simulink model "subsystems"  (R2023b)
settings: Solver=FixedStepAuto  StartTime=0.0  StopTime=10.0  FixedStep=1e-3  RelTol=1e-3
libraries: simulink x5
settings Model: Creator=DELL  LastModifiedBy=DELL

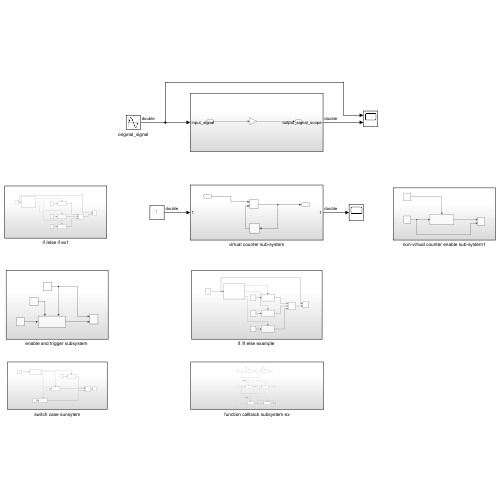
[thumbnail: Simulink's stored preview of the top-level diagram]
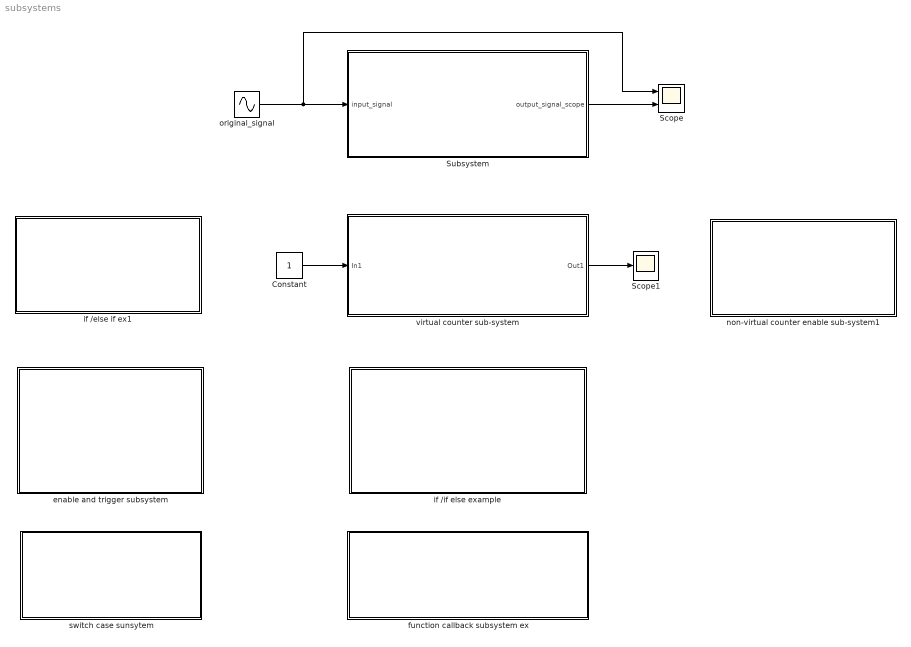
== system subsystems ==
  Constant : Constant
  Scope : Scope  NumInputPorts=2
  Scope1 : Scope
  Subsystem : Subsystem
  "enable and trigger subsystem " : Subsystem
  function callback subsystem ex : Subsystem
  if /else if ex1 : Subsystem
  "if /if else example " : Subsystem
  non-virtual counter enable sub-system1 : Subsystem
  original_signal : Sin  SampleTime=0
  switch case sunsytem : Subsystem
  virtual counter sub-system : Subsystem
  wires:
  original_signal/1 -> Subsystem/1(input_signal), Scope/1
  Subsystem/1(output_signal_scope) -> Scope/2
  Constant/1 -> virtual counter sub-system/1(In1)
  virtual counter sub-system/1(Out1) -> Scope1/1

== system subsystems/Subsystem ==
  input_signal : Inport
  Gain : Gain  Gain=2
  output_signal_scope : Outport
  wires:
  input_signal/1 -> Gain/1
  Gain/1 -> output_signal_scope/1

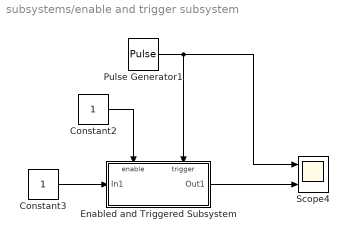
== system subsystems/enable and trigger subsystem  ==
  Constant2 : Constant
  Constant3 : Constant
  Enabled and Triggered Subsystem : Subsystem  TreatAsAtomicUnit=on
  Pulse Generator1 : DiscretePulseGenerator  PulseType=Time based  PulseWidth=50
  Scope4 : Scope  NumInputPorts=2
  wires:
  Pulse Generator1/1 -> Enabled and Triggered Subsystem/Trigger, Scope4/1
  Constant3/1 -> Enabled and Triggered Subsystem/1(In1)
  Constant2/1 -> Enabled and Triggered Subsystem/Enable
  Enabled and Triggered Subsystem/1(Out1) -> Scope4/2

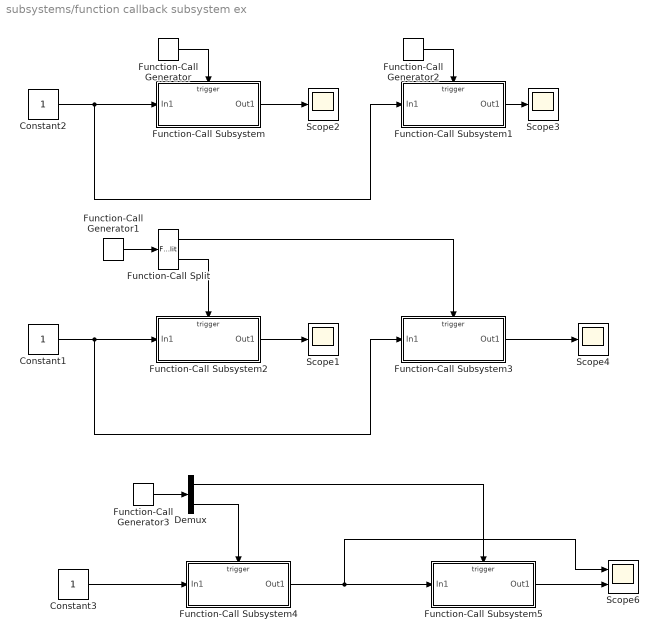
== system subsystems/function callback subsystem ex ==
  Constant1 : Constant
  Constant2 : Constant
  Constant3 : Constant
  Demux : Demux  Outputs=2
  Function-Call Generator : simulink/Ports & Subsystems/Function-Call Generator  sample_time=0.25  numberOfIterations=1  DisallowWideOutput=off
  Function-Call Generator1 : simulink/Ports & Subsystems/Function-Call Generator  sample_time=0.25  numberOfIterations=1  DisallowWideOutput=off
  Function-Call Generator2 : simulink/Ports & Subsystems/Function-Call Generator  sample_time=0.25  numberOfIterations=1  DisallowWideOutput=off
  Function-Call Generator3 : simulink/Ports & Subsystems/Function-Call Generator  sample_time=1  numberOfIterations=1  DisallowWideOutput=off
  Function-Call Split : FunctionCallSplit  IconShape=distinctive  NumOutputPorts=2  OutputPortLayout=default
  Function-Call Subsystem : Subsystem  TreatAsAtomicUnit=on
  Function-Call Subsystem1 : Subsystem  TreatAsAtomicUnit=on
  Function-Call Subsystem2 : Subsystem  TreatAsAtomicUnit=on
  Function-Call Subsystem3 : Subsystem  TreatAsAtomicUnit=on
  Function-Call Subsystem4 : Subsystem  TreatAsAtomicUnit=on
  Function-Call Subsystem5 : Subsystem  TreatAsAtomicUnit=on
  Scope{1..4} (4 alike) : Scope
  Scope6 : Scope  NumInputPorts=2
  wires:
  Function-Call Subsystem/1(Out1) -> Scope2/1
  Function-Call Generator/1 -> Function-Call Subsystem/Trigger
  Constant2/1 -> Function-Call Subsystem1/1(In1), Function-Call Subsystem/1(In1)
  Function-Call Subsystem1/1(Out1) -> Scope3/1
  Function-Call Generator2/1 -> Function-Call Subsystem1/Trigger
  Function-Call Subsystem3/1(Out1) -> Scope4/1
  Constant1/1 -> Function-Call Subsystem2/1(In1), Function-Call Subsystem3/1(In1)
  Function-Call Subsystem2/1(Out1) -> Scope1/1
  Function-Call Generator1/1 -> Function-Call Split/1
  Function-Call Split/2 -> Function-Call Subsystem2/Trigger
  Function-Call Split/1 -> Function-Call Subsystem3/Trigger
  Demux/1 -> Function-Call Subsystem5/Trigger
  Demux/2 -> Function-Call Subsystem4/Trigger
  Function-Call Generator3/1 -> Demux/1
  Function-Call Subsystem4/1(Out1) -> Function-Call Subsystem5/1(In1), Scope6/1
  Constant3/1 -> Function-Call Subsystem4/1(In1)
  Function-Call Subsystem5/1(Out1) -> Scope6/2

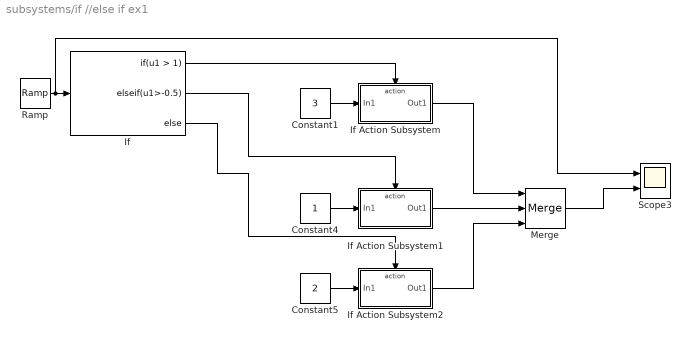
== system subsystems/if //else if ex1 ==
  Constant1 : Constant  Value=3
  Constant4 : Constant
  Constant5 : Constant  Value=2
  If : If  IfExpression=u1 > 1  ElseIfExpressions=u1>-0.5
  If Action Subsystem : Subsystem  TreatAsAtomicUnit=on
  If Action Subsystem1 : Subsystem  TreatAsAtomicUnit=on
  If Action Subsystem2 : Subsystem  TreatAsAtomicUnit=on
  Merge : Merge  Inputs=3
  Ramp : simulink/Sources/Ramp  slope=1  start=0  InitialOutput=-0.5
  Scope3 : Scope  NumInputPorts=2
  wires:
  If Action Subsystem/1(Out1) -> Merge/1
  Ramp/1 -> Scope3/1, If/1
  If/1 -> If Action Subsystem/Action
  Constant4/1 -> If Action Subsystem1/1(In1)
  Merge/1 -> Scope3/2
  If Action Subsystem2/1(Out1) -> Merge/3
  If/3 -> If Action Subsystem2/Action
  If/2 -> If Action Subsystem1/Action
  Constant1/1 -> If Action Subsystem/1(In1)
  Constant5/1 -> If Action Subsystem2/1(In1)
  If Action Subsystem1/1(Out1) -> Merge/2

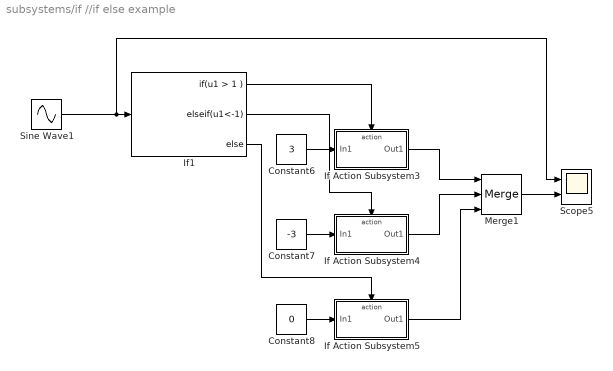
== system subsystems/if //if else example  ==
  Constant6 : Constant  Value=3
  Constant7 : Constant  Value=-3
  Constant8 : Constant  Value=0
  If Action Subsystem3 : Subsystem  TreatAsAtomicUnit=on
  If Action Subsystem4 : Subsystem  TreatAsAtomicUnit=on
  If Action Subsystem5 : Subsystem  TreatAsAtomicUnit=on
  If1 : If  IfExpression=u1 > 1  ElseIfExpressions=u1<-1
  Merge1 : Merge  Inputs=3
  Scope5 : Scope  NumInputPorts=2
  Sine Wave1 : Sin  Amplitude=7  SampleTime=0
  wires:
  If1/1 -> If Action Subsystem3/Action
  If Action Subsystem3/1(Out1) -> Merge1/1
  Merge1/1 -> Scope5/2
  If1/2 -> If Action Subsystem4/Action
  If Action Subsystem4/1(Out1) -> Merge1/2
  Constant7/1 -> If Action Subsystem4/1(In1)
  Sine Wave1/1 -> Scope5/1, If1/1
  Constant6/1 -> If Action Subsystem3/1(In1)
  Constant8/1 -> If Action Subsystem5/1(In1)
  If Action Subsystem5/1(Out1) -> Merge1/3
  If1/3 -> If Action Subsystem5/Action

== system subsystems/non-virtual counter enable sub-system1 ==
  Pulse Generator : DiscretePulseGenerator  PulseType=Time based  Period=1  PulseWidth=50
  Scope2 : Scope  NumInputPorts=2
  Sine Wave : Sin  SampleTime=0
  non-virtual counter enable sub-system : Subsystem  TreatAsAtomicUnit=on
  wires:
  Sine Wave/1 -> Scope2/2, non-virtual counter enable sub-system/1(In1)
  Pulse Generator/1 -> non-virtual counter enable sub-system/Enable
  non-virtual counter enable sub-system/1(Out1) -> Scope2/1

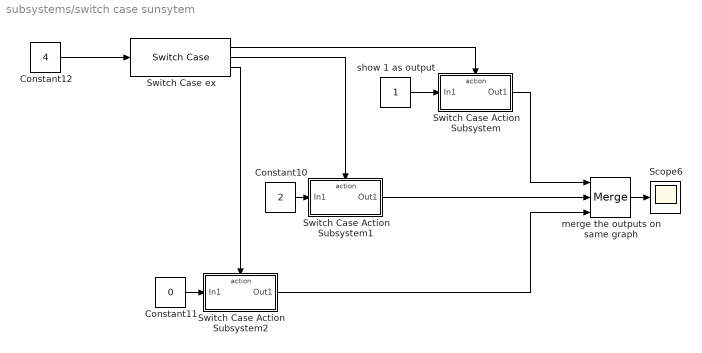
== system subsystems/switch case sunsytem ==
  Constant10 : Constant  Value=2
  Constant11 : Constant  Value=0
  Constant12 : Constant  Value=4
  Scope6 : Scope
  Switch Case Action Subsystem : Subsystem  TreatAsAtomicUnit=on
  Switch Case Action Subsystem1 : Subsystem  TreatAsAtomicUnit=on
  Switch Case Action Subsystem2 : Subsystem  TreatAsAtomicUnit=on
  Switch Case ex : SwitchCase  CaseConditions={1,[2,3,5]}
  "merge the outputs on same graph " : Merge  Inputs=3
  "show 1 as output " : Constant
  wires:
  Constant12/1 -> Switch Case ex/1
  Switch Case Action Subsystem1/1(Out1) -> "merge the outputs on same graph "/2
  Switch Case ex/2 -> Switch Case Action Subsystem1/Action
  "show 1 as output "/1 -> Switch Case Action Subsystem/1(In1)
  Switch Case ex/3 -> Switch Case Action Subsystem2/Action
  Switch Case ex/1 -> Switch Case Action Subsystem/Action
  Constant11/1 -> Switch Case Action Subsystem2/1(In1)
  Switch Case Action Subsystem/1(Out1) -> "merge the outputs on same graph "/1
  "merge the outputs on same graph "/1 -> Scope6/1
  Constant10/1 -> Switch Case Action Subsystem1/1(In1)
  Switch Case Action Subsystem2/1(Out1) -> "merge the outputs on same graph "/3

== system subsystems/virtual counter sub-system ==
  In1 : Inport
  Add : Sum
  Unit Delay : UnitDelay  SampleTime=-1  HasFrameUpgradeWarning=on
  Out1 : Outport
  wires:
  Add/1 -> Out1/1, Unit Delay/1
  Unit Delay/1 -> Add/2
  In1/1 -> Add/1

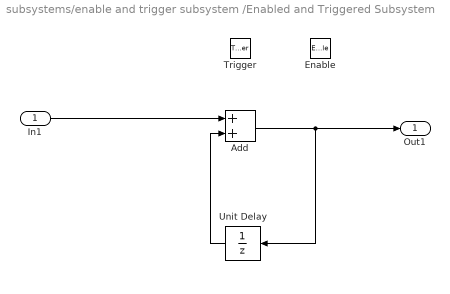
== system subsystems/enable and trigger subsystem /Enabled and Triggered Subsystem ==
  In1 : Inport
  Enable : EnablePort
  Trigger : TriggerPort  TriggerType=either  VariantControl=(inherit)
  Add : Sum
  Unit Delay : UnitDelay  SampleTime=-1  HasFrameUpgradeWarning=on
  Out1 : Outport
  wires:
  In1/1 -> Add/1
  Unit Delay/1 -> Add/2
  Add/1 -> Unit Delay/1, Out1/1

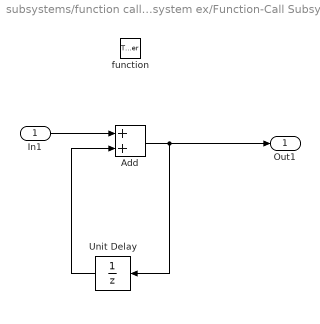
== system subsystems/function callback subsystem ex/Function-Call Subsystem ==
  In1 : Inport
  function : TriggerPort  TriggerType=function-call  VariantControl=(inherit)
  Add : Sum
  Unit Delay : UnitDelay  SampleTime=-1  HasFrameUpgradeWarning=on
  Out1 : Outport
  wires:
  In1/1 -> Add/1
  Unit Delay/1 -> Add/2
  Add/1 -> Unit Delay/1, Out1/1

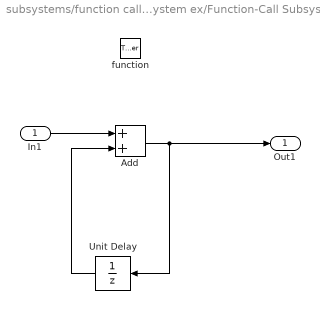
== system subsystems/function callback subsystem ex/Function-Call Subsystem1 ==
  In1 : Inport
  function : TriggerPort  TriggerType=function-call  VariantControl=(inherit)
  Add : Sum
  Unit Delay : UnitDelay  SampleTime=-1  HasFrameUpgradeWarning=on
  Out1 : Outport
  wires:
  Add/1 -> Out1/1, Unit Delay/1
  Unit Delay/1 -> Add/2
  In1/1 -> Add/1

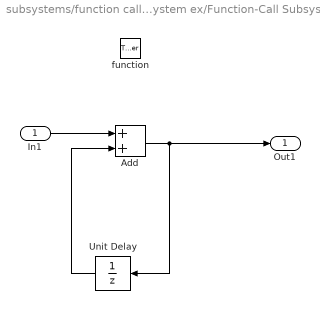
== system subsystems/function callback subsystem ex/Function-Call Subsystem2 ==
  In1 : Inport
  function : TriggerPort  TriggerType=function-call  VariantControl=(inherit)
  Add : Sum
  Unit Delay : UnitDelay  SampleTime=-1  HasFrameUpgradeWarning=on
  Out1 : Outport
  wires:
  Add/1 -> Out1/1, Unit Delay/1
  Unit Delay/1 -> Add/2
  In1/1 -> Add/1

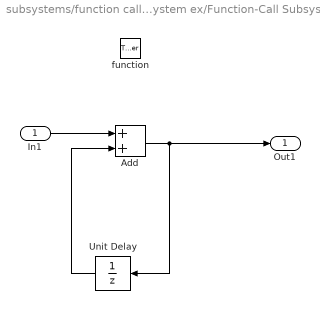
== system subsystems/function callback subsystem ex/Function-Call Subsystem3 ==
  In1 : Inport
  function : TriggerPort  TriggerType=function-call  VariantControl=(inherit)
  Add : Sum
  Unit Delay : UnitDelay  SampleTime=-1  HasFrameUpgradeWarning=on
  Out1 : Outport
  wires:
  In1/1 -> Add/1
  Unit Delay/1 -> Add/2
  Add/1 -> Unit Delay/1, Out1/1

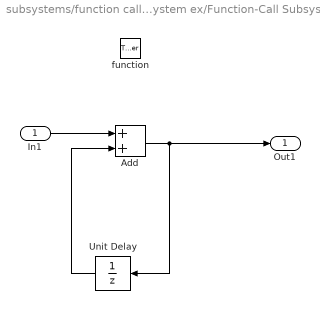
== system subsystems/function callback subsystem ex/Function-Call Subsystem4 ==
  In1 : Inport
  function : TriggerPort  TriggerType=function-call  VariantControl=(inherit)
  Add : Sum
  Unit Delay : UnitDelay  SampleTime=-1  HasFrameUpgradeWarning=on
  Out1 : Outport
  wires:
  In1/1 -> Add/1
  Unit Delay/1 -> Add/2
  Add/1 -> Unit Delay/1, Out1/1

== system subsystems/function callback subsystem ex/Function-Call Subsystem5 ==
  In1 : Inport
  function : TriggerPort  TriggerType=function-call  VariantControl=(inherit)
  Add : Sum
  Unit Delay : UnitDelay  SampleTime=-1  HasFrameUpgradeWarning=on
  Out1 : Outport
  wires:
  Add/1 -> Out1/1, Unit Delay/1
  Unit Delay/1 -> Add/2
  In1/1 -> Add/1

== system subsystems/if //else if ex1/If Action Subsystem ==
  In1 : Inport
  Action Port : ActionPort  ActionPortLabel=if(u1 > 1)
  Out1 : Outport
  wires:
  In1/1 -> Out1/1

== system subsystems/if //else if ex1/If Action Subsystem1 ==
  In1 : Inport
  Action Port : ActionPort  ActionPortLabel=elseif(u1>-0.5)
  Out1 : Outport
  wires:
  In1/1 -> Out1/1

== system subsystems/if //else if ex1/If Action Subsystem2 ==
  In1 : Inport
  Action Port : ActionPort  ActionPortLabel=else
  Out1 : Outport
  wires:
  In1/1 -> Out1/1

== system subsystems/if //if else example /If Action Subsystem3 ==
  In1 : Inport
  Action Port : ActionPort  ActionPortLabel=if(u1 > 1 )
  Out1 : Outport
  wires:
  In1/1 -> Out1/1

== system subsystems/if //if else example /If Action Subsystem4 ==
  In1 : Inport
  Action Port : ActionPort  ActionPortLabel=elseif(u1<-1)
  Out1 : Outport
  wires:
  In1/1 -> Out1/1

== system subsystems/if //if else example /If Action Subsystem5 ==
  In1 : Inport
  Action Port : ActionPort  ActionPortLabel=else
  Out1 : Outport
  wires:
  In1/1 -> Out1/1

== system subsystems/non-virtual counter enable sub-system1/non-virtual counter enable sub-system ==
  note: counter loop
  In1 : Inport
  Enable : EnablePort
  Add : Sum  Commented=on
  Unit Delay : UnitDelay  Commented=on  SampleTime=-1  HasFrameUpgradeWarning=on
  Out1 : Outport
  wires:
  Add/1 -> Unit Delay/1
  Unit Delay/1 -> Add/2
  In1/1 -> Out1/1

== system subsystems/switch case sunsytem/Switch Case Action Subsystem ==
  In1 : Inport
  Action Port : ActionPort  ActionPortLabel=case [ 1 ]:
  Out1 : Outport
  wires:
  In1/1 -> Out1/1

== system subsystems/switch case sunsytem/Switch Case Action Subsystem1 ==
  In1 : Inport
  Action Port : ActionPort  ActionPortLabel=case [ 2 3 5 ]:
  Out1 : Outport
  wires:
  In1/1 -> Out1/1

== system subsystems/switch case sunsytem/Switch Case Action Subsystem2 ==
  In1 : Inport
  Action Port : ActionPort  ActionPortLabel=default:
  Out1 : Outport
  wires:
  In1/1 -> Out1/1
